simulink library "lib_affectiveChar_behavior"  (R2014a)
settings: Solver=ode45  StartTime=0.0  StopTime=10.0  RelTol=1e-3
libraries: simulink x5
(part 2 of 4)

== stateflow chart lib_affectiveChar_behavior/boredPoseBrad ==
  state sendBML(arg) [function]
  state stateBoredPose
    entry:
    coping=0;
    boredPose(randi([1,6]));
    sendBML(  boredPose(randi([1,6])) );
  data: arg function_input double size=[256 1]; bmlID function_input double size=1; poseBML function_output double size=256; coping data_store_memory size=1
  function poseBML=boredPose(bmlID):
    | function poseBML=boredPose(bmlID)
    | 
    | aVarTruthTableCondition_1 = false;
    | aVarTruthTableCondition_2 = false;
    | aVarTruthTableCondition_3 = false;
    | aVarTruthTableCondition_4 = false;
    | aVarTruthTableCondition_5 = false;
    | aVarTruthTableCondition_6 = false;
    | aVarTruthTableCondition_7 = false;
    | aVarTruthTableCondition_8 = false;
    | 
    | 
    | 
    | aVarTruthTableCondition_1 = logical(bmlID==1);
    | 
    | 
    | aVarTruthTableCondition_2 = logical(bmlID==2);
    | 
    | 
    | aVarTruthTableCondition_3 = logical(bmlID==3);
    | 
    | 
    | aVarTruthTableCondition_4 = logical(bmlID==4);
    | 
    | 
    | aVarTruthTableCondition_5 = logical(bmlID==5);
    | 
    | 
    | aVarTruthTableCondition_6 = logical(bmlID==6);
    | 
    | 
    | aVarTruthTableCondition_7 = logical(bmlID==7);
    | 
    | 
    | aVarTruthTableCondition_8 = logical(bmlID==8);
    | 
    | if (aVarTruthTableCondition_1)
    |     aFcnTruthTableAction_1();
    | elseif (aVarTruthTableCondition_2)
    |     aFcnTruthTableAction_2();
    | elseif (aVarTruthTableCondition_3)
    |     aFcnTruthTableAction_3();
    | elseif (aVarTruthTableCondition_4)
    |     aFcnTruthTableAction_4();
    | elseif (aVarTruthTableCondition_5)
    |     aFcnTruthTableAction_5();
    | elseif (aVarTruthTableCondition_6)
    |     aFcnTruthTableAction_6();
    | elseif (aVarTruthTableCondition_7)
    |     aFcnTruthTableAction_3();
    | elseif (aVarTruthTableCondition_8)
    |     aFcnTruthTableAction_5();
    | else % Default
    |     aFcnTruthTableAction_3();
    | end
    | 
    | function aFcnTruthTableAction_1()
    | 
    | % ArmStretch
    | 
    | poseBML=encStr2Arr('<?xml version="1.0" ?><act><bml><animation name="ChrBrad@Idle01_ArmStretch01"/></bml></act>')
    | 
    | function aFcnTruthTableAction_2()
    | 
    | % Idle01_ToIdle03
    | 
    | poseBML=encStr2Arr('<?xml version="1.0" ?><act><bml><animation name="ChrBrad@Idle01_ToIdle03"/></bml></act>')
    | 
    | function aFcnTruthTableAction_3()
    | 
    | % WeightShift
    | 
    | poseBML=encStr2Arr('<?xml version="1.0" ?><act><bml><animation name="ChrBrad@Idle01_WeightShift01"/></bml></act>')
    | 
    | function aFcnTruthTableAction_4()
    | 
    | % ScratchChest
    | 
    | poseBML=encStr2Arr('<?xml version="1.0" ?><act><bml><animation name="ChrBrad@Idle01_ScratchChest01"/></bml></act>')
    | 
    | function aFcnTruthTableAction_5()
    | 
    | % ScratchHead
    | 
    | poseBML=encStr2Arr('<?xml version="1.0" ?><act><bml><animation name="ChrBrad@Idle01_ScratchHeadLf01"/></bml></act>')
    | 
    | function aFcnTruthTableAction_6()
    | 
    | % ShoulderStretch
    | 
    | poseBML=encStr2Arr('<?xml version="1.0" ?><act><bml><animation name="ChrBrad@Idle01_ShoulderStretch01"/></bml></act>')

== stateflow chart lib_affectiveChar_behavior/gazeAtUserBrad/createGazePawn ==
  state sendSBM(arg) [function]
  state sendBML(arg) [function]
  state idle
  state stateCreatePawn
    entry:
    sendSBM( encStr2Arr( 'gt = scene.createPawn("gazeTarget")' ) );
  state stateGazeatUser
    entry:
    sendBML(encStr2Arr('<?xml version="1.0" ?><act><bml><gaze sbm:joint-range="EYES NECK" target="gazeTarget"/></bml></act>'));
  (default) -> idle
  idle -> stateCreatePawn : after(3, sec)
  stateCreatePawn -> stateGazeatUser : after(1, sec)
  data: arg function_input double size=[256 1]; arg function_input double size=[256 1]

== stateflow chart lib_affectiveChar_behavior/smile ==
  note: Agent may smile when posing but does not smile when avert head.
  state stateInitial
    entry: avert=0;
  state sendBML(arg) [function]
  state stateCheck
  note: num of bmlID=2
  state stateSmile
    entry: isPosing=1;
    sendBML( smileTable(1) );
  (default) -> stateInitial
  stateInitial -> stateCheck
  stateSmile -> stateCheck [order 1] : [([isSmiling==0])||([avert~=0])]
  stateCheck -> stateSmile : [([isSmiling==1])&([avert==0])]
  stateSmile -> stateSmile [order 2]
  data: arg function_input double size=[256 1]; bmlID function_input double; poseBML function_output double size=[256,1]; isPosing data_store_memory size=2; isSmiling input double size=1 =0; avert data_store_memory =0
  function poseBML = smileTable(bmlID):
    | function poseBML = smileTable(bmlID)
    | 
    | aVarTruthTableCondition_1 = false;
    | aVarTruthTableCondition_2 = false;
    | 
    | 
    | % smile
    | 
    | aVarTruthTableCondition_1 = logical(bmlID==1);
    | 
    | % neutralHeadGaze
    | 
    | aVarTruthTableCondition_2 = logical(bmlID==2);
    | 
    | if (aVarTruthTableCondition_1)
    |     aFcnTruthTableAction_1();
    | elseif (aVarTruthTableCondition_2)
    |     aFcnTruthTableAction_2();
    | else % Default
    |     aFcnTruthTableAction_1();
    | end
    | 
    | function aFcnTruthTableAction_1()
    | 
    | % smile
    | 
    | poseBML=encStr2Arr('<?xml version="1.0" ?><act><bml><face amount="1" au="12" end="8" relax="6" side="BOTH" start="0" stroke="3" type="facs"/><face amount="0.5" au="6" end="8" relax="6" side="BOTH" start="0" stroke="3" type="facs"/></bml></act>');
    | 
    | function aFcnTruthTableAction_2()
    | 
    | % neutralHeadGaze
    | 
    | poseBML=encStr2Arr('<?xml version="1.0" ?><act><bml><gaze target="camera" sbm:time-hint="0.2"/></bml></act>');

== stateflow chart lib_affectiveChar_behavior/sendEmotionBMLs ==
  state stateFacialExpression
    entry:
    EAU(externalE)
    sendBML(cmdBML_AUs(EAU(externalE)));
  state sendBML(arg) [function]
  (default) -> stateFacialExpression
  stateFacialExpression -> stateFacialExpression : after(1,secs)
  data: arg function_input double size=[256 1]; E function_input; AU function_output uint32; externalE input double size=1 =5
  events: secs input RISING_EDGE_EVENT
  function AU=EAU(E):
    | function AU=EAU(E)
    | 
    | aVarTruthTableCondition_1 = false;
    | aVarTruthTableCondition_2 = false;
    | aVarTruthTableCondition_3 = false;
    | aVarTruthTableCondition_4 = false;
    | aVarTruthTableCondition_5 = false;
    | aVarTruthTableCondition_6 = false;
    | aVarTruthTableCondition_7 = false;
    | aVarTruthTableCondition_8 = false;
    | aVarTruthTableCondition_9 = false;
    | 
    | 
    | % , happy
    | 
    | aVarTruthTableCondition_1 = logical(E==1);
    | 
    | % , excited
    | 
    | aVarTruthTableCondition_2 = logical(E==2);
    | 
    | % , fear
    | 
    | aVarTruthTableCondition_3 = logical(E==3);
    | 
    | % , frustration
    | 
    | aVarTruthTableCondition_4 = logical(E==4);
    | 
    | % , neutral
    | 
    | aVarTruthTableCondition_5 = logical(E==5);
    | 
    | % , contempt
    | 
    | aVarTruthTableCondition_6 = logical(E==6);
    | 
    | % , bored
    | 
    | aVarTruthTableCondition_7 = logical(E==7);
    | 
    | % , sad
    | 
    | aVarTruthTableCondition_8 = logical(E==8);
    | 
    | % , angry
    | 
    | aVarTruthTableCondition_9 = logical(E==9);
    | 
    | if (aVarTruthTableCondition_1)
    |     aFcnTruthTableAction_1();
    | elseif (aVarTruthTableCondition_2)
    |     aFcnTruthTableAction_2();
    | elseif (aVarTruthTableCondition_3)
    |     aFcnTruthTableAction_3();
    | elseif (aVarTruthTableCondition_4)
    |     aFcnTruthTableAction_4();
    | elseif (aVarTruthTableCondition_5)
    |     aFcnTruthTableAction_5();
    | elseif (aVarTruthTableCondition_6)
    |     aFcnTruthTableAction_6();
    | elseif (aVarTruthTableCondition_7)
    |     aFcnTruthTableAction_7();
    | elseif (aVarTruthTableCondition_8)
    |     aFcnTruthTableAction_8();
    | elseif (aVarTruthTableCondition_9)
    |     aFcnTruthTableAction_9();
    | else % Default
    |     aFcnTruthTableAction_5();
    | end
    | 
    | function aFcnTruthTableAction_1()
    | 
    | % action unit
    | 
    | AU=[6,12,142];
    | 
    | function aFcnTruthTableAction_2()
    | 
    | 
    | AU=[1,2,144];
    | 
    | function aFcnTruthTableAction_3()
    | 
    | 
    | AU=[1,2,4,20,26,386];
    | 
    | function aFcnTruthTableAction_4()
    | 
    | 
    | AU=[1,2,144];
    | 
    | function aFcnTruthTableAction_5()
    | 
    | 
    | AU=[6,12,142];
    | 
    | function aFcnTruthTableAction_6()
    | 
    | 
    | AU=[12,14,143];
    | 
    | function aFcnTruthTableAction_7()
    | 
    | 
    | AU=[6,12,142];
    | 
    | function aFcnTruthTableAction_8()
    | 
    | 
    | AU=[1,4,15,180];
    | 
    | function aFcnTruthTableAction_9()
    | 
    | 
    | AU=[4,5,7,10,23,26,410];

== matlab function lib_affectiveChar_behavior/gazeAtUserBrad/gazeControl/movePawn ==
  data: x input; y input; arrBML output
function arrBML   = fcn( x,y )
coder.extrinsic('sprintf')
%for agent to gaze at the user, we create a pawn where user stands and agent gazes at the pawn
%1) AnTS: x btw 200,600/gaze btw 0,1
 x=(x-200)/400;
c = countDigits(x);

mystr=blanks(66+c);
%mystr = sprintf('scene.getPawn(\"gazeTarget\").setPosition(SrVec(%d, %d ,%d))',x,0,150);
mystr = sprintf('scene.getPawn(\"gazeTarget\").setPosition(SrVec(%0.1f , %d ,%d))',x,1.7,2); %x btw 0,1
arrBML = encStr2Arr(mystr);

end

== stateflow chart lib_affectiveChar_behavior/copingBrad ==
  state sendBML(arg) [function]
  state stateCoping
    entry:
    sendBML( copingInvaded(randi([1,4])) );
  data: arg function_input double size=[256 1]; bmlID function_input double size=1; invadedBML function_output double size=256
  function invadedBML=copingInvaded(bmlID):
    | function invadedBML=copingInvaded(bmlID)
    | 
    | aVarTruthTableCondition_1 = false;
    | aVarTruthTableCondition_2 = false;
    | aVarTruthTableCondition_3 = false;
    | aVarTruthTableCondition_4 = false;
    | 
    | 
    | 
    | aVarTruthTableCondition_1 = logical(bmlID==1);
    | 
    | 
    | aVarTruthTableCondition_2 = logical(bmlID==2);
    | 
    | 
    | aVarTruthTableCondition_3 = logical(bmlID==3);
    | 
    | 
    | aVarTruthTableCondition_4 = logical(bmlID==4);
    | 
    | if (aVarTruthTableCondition_1)
    |     aFcnTruthTableAction_1();
    | elseif (aVarTruthTableCondition_2)
    |     aFcnTruthTableAction_2();
    | elseif (aVarTruthTableCondition_3)
    |     aFcnTruthTableAction_3();
    | elseif (aVarTruthTableCondition_4)
    |     aFcnTruthTableAction_4();
    | else % Default
    |     aFcnTruthTableAction_4();
    | end
    | 
    | function aFcnTruthTableAction_1()
    | 
    | % Scratch
    | 
    | invadedBML=encStr2Arr('<?xml version="1.0" ?><act><bml><animation name="ChrBrad@Idle01_ScratchTempleLf01"/><face type="FACS" side="right" au="4" amount="1.5" start="0" end="5" /></bml></act>')
    | 
    | function aFcnTruthTableAction_2()
    | 
    | % Scared-b
    | 
    | invadedBML=encStr2Arr('<?xml version="1.0" ?><act><bml><face type="FACS" side="BOTH" au="1" amount="1" start="0" end="5" /><face type="FACS" side="BOTH" au="2" amount="1" start="0" end="5" /></bml></act>')
    | 
    | function aFcnTruthTableAction_3()
    | 
    | % frown-b
    | 
    | invadedBML=encStr2Arr('<?xml version="1.0" ?><act><bml><face type="FACS" side="BOTH" au="4" amount="1.5" start="0" end="5" /></bml></act>')
    | 
    | function aFcnTruthTableAction_4()
    | 
    | % frown-hand
    | 
    | invadedBML=encStr2Arr('<?xml version="1.0" ?><act><bml><animation name="ChrBrad@Idle01_ToIdle03"/><face type="FACS" side="right" au="2" amount="1.5" start="0" end="5" /><face type="FACS" side="right" au="4" amount="1.5" start="0" end="5" /></bml></act>')

== matlab function lib_affectiveChar_behavior/calculateAgentValenceArousal/VAEmotion ==
  data: V input; e output; A input double
function e = fcn(V, A)

aVarTruthTableCondition_1 = false;
aVarTruthTableCondition_2 = false;
aVarTruthTableCondition_3 = false;
aVarTruthTableCondition_4 = false;
aVarTruthTableCondition_5 = false;
aVarTruthTableCondition_6 = false;
aVarTruthTableCondition_7 = false;
aVarTruthTableCondition_8 = false;
aVarTruthTableCondition_9 = false;


% valence and arousal

aVarTruthTableCondition_1 = logical(V==2 && A==1);


aVarTruthTableCondition_2 = logical(V==2 && A==2);


aVarTruthTableCondition_3 = logical(V==-1 && A==2);


aVarTruthTableCondition_4 = logical(V==-2 && A==1);


aVarTruthTableCondition_5 = logical(V==2 && A==-1);


aVarTruthTableCondition_6 = logical(V==1 && A==-2);


aVarTruthTableCondition_7 = logical(V==-1 && A==-2);


aVarTruthTableCondition_8 = logical(V==-2 && A==-1);


aVarTruthTableCondition_9 = logical(A==1.5 && V==-1.5);

if (aVarTruthTableCondition_1)
    aFcnTruthTableAction_1();
elseif (aVarTruthTableCondition_2)
    aFcnTruthTableAction_2();
elseif (aVarTruthTableCondition_3)
    aFcnTruthTableAction_3();
elseif (aVarTruthTableCondition_4)
    aFcnTruthTableAction_4();
elseif (aVarTruthTableCondition_5)
    aFcnTruthTableAction_5();
elseif (aVarTruthTableCondition_6)
    aFcnTruthTableAction_6();
elseif (aVarTruthTableCondition_7)
    aFcnTruthTableAction_7();
elseif (aVarTruthTableCondition_8)
    aFcnTruthTableAction_8();
elseif (aVarTruthTableCondition_9)
    aFcnTruthTableAction_9();
else % Default
    aFcnTruthTableAction_5();
end

function aFcnTruthTableAction_1()

% emotion-happy

e=1;

function aFcnTruthTableAction_2()

% exite

e=2;

function aFcnTruthTableAction_3()

% fear

e=3;

function aFcnTruthTableAction_4()

% frustration

e=4;

function aFcnTruthTableAction_5()

% idle

e=5;

function aFcnTruthTableAction_6()

% contempt

e=6;

function aFcnTruthTableAction_7()

% bored

e=7;

function aFcnTruthTableAction_8()

% sad

e=8;

function aFcnTruthTableAction_9()

% anger

e=9;
